simulink model "msfcndemo_varsize"  (Simulink 7.6)
settings: Solver=FixedStepDiscrete  StartTime=0.0  StopTime=2.0  FixedStep=0.2  RelTol=1e-3
libraries: simulink x1
settings Model: Creator=The MathWorks Inc.
settings DataIOCC: SaveFormat=StructureWithTime
settings OptimizationCC: EfficientMapNaN2IntZero=off

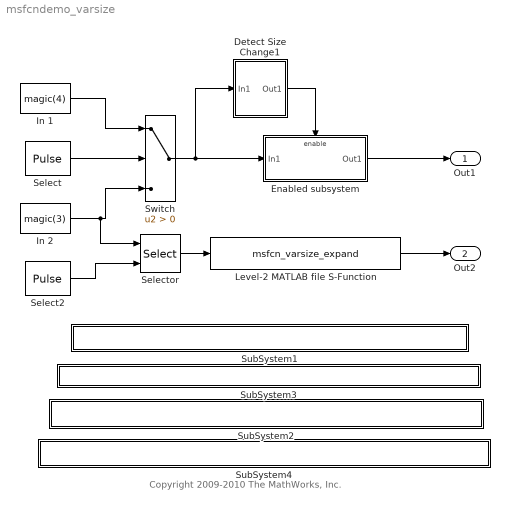
== system msfcndemo_varsize ==
  note: Copyright 2009-2010 The MathWorks, Inc.
  Detect Size Change1 : Subsystem
  Enabled subsystem : Subsystem  TreatAsAtomicUnit=on
  In 1 : Constant  Value=magic(4)
  In 2 : Constant  Value=magic(3)
  Level-2 MATLAB file S-Function : M-S-Function  FunctionName=msfcn_varsize_expand  Parameters=maxNumEls  mask(S-function:msfcn_holdStateUntilReset){maxNumEls=100}
      mask prompts: maxNumEls "Maximum number of elements"
      mask help: This is a level-2 MATLAB file S-function which demonstrates how to implement a block that holds its states until reset, when the size of the signal can change.
      mask Display: disp('Expand')
  Select : DiscretePulseGenerator  Period=8  PulseWidth=4  SampleTime=0.2
  Select2 : DiscretePulseGenerator  Period=8  PulseWidth=4  SampleTime=0.2
  Selector : Selector  NumberOfDimensions=2  IndexMode=Zero-based  InputPortWidth=3  IndexOptions=Index vector (dialog),Index vector (port)  Indices=1,1  OutputSizes=1,1
  SubSystem1 : Subsystem  mask{filename=msfcn_varsize_expand.m}
      mask init:
      | x=sfundemo_maskdisp;
      settings: AttributesFormatString=\n  OpenFcn=sfundemo_openfcn
      mask Display: disp(x);
  SubSystem2 : Subsystem  mask{filename=msfcn_varsize_holdStatesUntilReset.m}
      mask init:
      | x=sfundemo_maskdisp;
      settings: AttributesFormatString=\n  OpenFcn=sfundemo_openfcn
      mask Display: disp(x);
  SubSystem3 : Subsystem  mask{filename=msfcn_varsize_expand.tlc}
      mask init:
      | x=sfundemo_maskdisp;
      settings: AttributesFormatString=\n  OpenFcn=sfundemo_openfcn
      mask Display: disp(x);
  SubSystem4 : Subsystem  mask{filename=msfcn_varsize_holdStatesUntilReset.tlc}
      mask init:
      | x=sfundemo_maskdisp;
      settings: AttributesFormatString=\n  OpenFcn=sfundemo_openfcn
      mask Display: disp(x);
  Switch : Switch  Criteria=u2 > Threshold  AllowDiffInputSizes=on
  Out1 : Outport
  Out2 : Outport  Port=2
  wires:
  In 1/1 -> Switch/1
  Select/1 -> Switch/2
  In 2/1 -> Switch/3, Selector/1
  Switch/1 -> Enabled subsystem/1(In1), Detect Size Change1/1(In1)
  Enabled subsystem/1(Out1) -> Out1/1
  Detect Size Change1/1(Out1) -> Enabled subsystem/Enable
  Selector/1 -> Level-2 MATLAB file S-Function/1
  Level-2 MATLAB file S-Function/1 -> Out2/1
  Select2/1 -> Selector/2

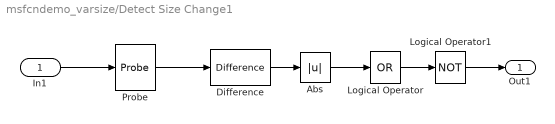
== system msfcndemo_varsize/Detect Size Change1 ==
  In1 : Inport
  Abs : Abs
  Difference : simulink/Discrete/Difference  SystemSampleTime=-1  ICPrevInput=0.0  OutMin=[]  OutMax=[]  OutDataType=fixdt(1, 16)  OutScaling=2^-10  DoSatur=off
  Logical Operator : Logic  Operator=OR  Inputs=1  AllPortsSameDT=off  OutDataTypeStr=boolean
  Logical Operator1 : Logic  Operator=NOT  Inputs=1  AllPortsSameDT=off  OutDataTypeStr=boolean
  Probe : Probe  ProbeWidth=off  ProbeSampleTime=off  ProbeComplexSignal=off  ProbeSignalDimensions=on
  Out1 : Outport
  wires:
  Logical Operator1/1 -> Out1/1
  Difference/1 -> Abs/1
  Probe/1 -> Difference/1
  In1/1 -> Probe/1
  Abs/1 -> Logical Operator/1
  Logical Operator/1 -> Logical Operator1/1

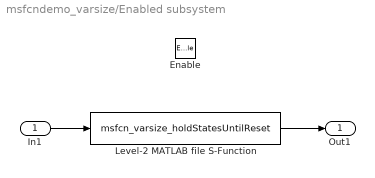
== system msfcndemo_varsize/Enabled subsystem ==
  In1 : Inport
  Enable : EnablePort  StatesWhenEnabling=reset
  Level-2 MATLAB file S-Function : M-S-Function  FunctionName=msfcn_varsize_holdStatesUntilReset
      mask Type: S-function:msfcn_holdStateUntilReset
      mask Description: This is a level-2 MATLAB file S-function which demonstrates how to implement a block that holds its states until reset, when the size of the signal can change.
      mask Display: disp('Hold States Until Reset')
  Out1 : Outport
  wires:
  In1/1 -> Level-2 MATLAB file S-Function/1
  Level-2 MATLAB file S-Function/1 -> Out1/1

== system msfcndemo_varsize/SubSystem1 ==

== system msfcndemo_varsize/SubSystem2 ==

== system msfcndemo_varsize/SubSystem3 ==

== system msfcndemo_varsize/SubSystem4 ==
